simulink model "gm_untitled"  (R2025a)
settings: Solver=VariableStepAuto  StartTime=0.0  StopTime=10.0  RelTol=1e-3
libraries: simulink x1
settings Model: Creator=HP  LastModifiedBy=HP
settings OptimizationCC: BlockReduction=off  ConditionallyExecuteInputs=off  DefaultParameterBehavior=Inlined
settings DebuggingCC: AlgebraicLoopMsg=error  InheritedTsInSrcMsg=none
settings HardwareCC: ProdBitPerPointer=32.0  ProdBitPerSizeT=32.0  ProdBitPerPtrDiffT=32.0  ProdLargestAtomicFloat=None  ProdIntDivRoundTo=Undefined  ProdEndianess=Unspecified  ProdWordSize=32.0  ProdHWDeviceType=ASIC/FPGA->ASIC/FPGA  TargetBitPerPointer=64.0  TargetBitPerSizeT=64.0  TargetBitPerPtrDiffT=64.0  TargetLongLongMode=on  TargetIntDivRoundTo=Zero  TargetEndianess=LittleEndian  TargetWordSize=64.0  TargetHWDeviceType=Custom Processor->MATLAB Host Computer  ProdEqTarget=off

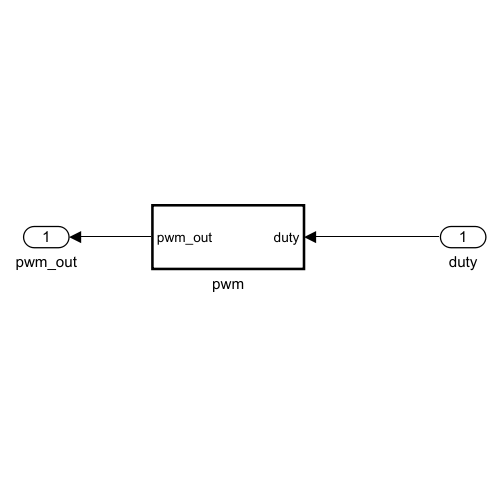
[thumbnail: Simulink's stored preview of the top-level diagram]
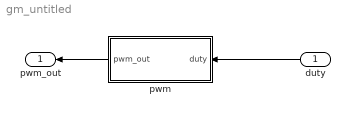
== system gm_untitled ==
  duty : Inport
  pwm : Subsystem  TreatAsAtomicUnit=on
  pwm_out : Outport
  wires:
  duty/1 -> pwm/1(duty)
  pwm/1(pwm_out) -> pwm_out/1

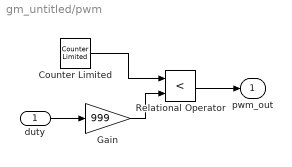
== system gm_untitled/pwm ==
  duty : Inport
  Counter Limited : simulink/Sources/Counter Limited  uplimit=999  tsamp=1e-6
  Gain : Gain  Gain=999  OutDataTypeStr=fixdt(1,16,0)
  Relational Operator : RelationalOperator  Operator=<  OutDataTypeStr=boolean  RndMeth=Simplest  InputSameDT=off
  pwm_out : Outport
  wires:
  Relational Operator/1 -> pwm_out/1
  duty/1 -> Gain/1
  Gain/1 -> Relational Operator/2
  Counter Limited/1 -> Relational Operator/1
